simulink model "Acceleration_R2016a"  (Simulink 8.7)
settings: Solver=VariableStepAuto  SolverMode=SingleTasking  StartTime=0.0  StopTime=30  FixedStep=0.1  RelTol=1e-3
values from neighbouring files (symbols this model uses):
  a = 31.111    [variabeln.m]
  b = -12.44444    [variabeln.m]
  Fz0 = 400*g    (= 3924)    [variabeln.m]
  g = 9.81    [variabeln.m]
  gear_ratio = 7.13    [variabeln.m]
  h_CoM = 0.5    [variabeln.m]
  J = 1    [variabeln.m]
  K_lqr = lqr(A,B,Q,R)    [variabeln.m]
  l = l_f+l_r    (= 3)    [variabeln.m]
  l_f = 1.5    [variabeln.m]
  lambda_target = 0.1    [variabeln.m]
  m = 700    [variabeln.m]
  Q = 100    [variabeln.m]
  R = 0.01    [variabeln.m]
  r = 0.25    [variabeln.m]
  saturation_voltage_high = 4.9    [variabeln.m]
  saturation_voltage_low = 0.4    [variabeln.m]
  Ta0 = 800    [variabeln.m]
  theta1 = 0.86    [variabeln.m]
  theta2 = 33.82    [variabeln.m]
  theta3 = 0.35    [variabeln.m]
  W_luft = 0.5*cw*A*rho    (= 0.45)    [variabeln.m]
libraries: simulink x1
settings Model: Creator=frede  LastModifiedBy=Dominic
settings DataIOCC: ExternalInput=[t, u,m,g,r,J,theta1,theta2,theta3,v0,gear_ratio,v_max]  LimitDataPoints=off  SaveFormat=Dataset
settings DebuggingCC: UnderspecifiedInitializationDetection=Simplified  MergeDetectMultiDrivingBlocksExec=error  MaxConsecutiveZCsMsg=none  SFUnexpectedBacktrackingDiag=error  SFNoUnconditionalDefaultTransitionDiag=error
settings HardwareCC: ProdBitPerPointer=64  ProdLargestAtomicFloat=Float  ProdIntDivRoundTo=Zero  ProdEndianess=LittleEndian  ProdWordSize=64  ProdHWDeviceType=Intel->x86-64 (Windows64)
settings ModelReferenceCC: PropagateSignalLabelsOutOfModel=on
settings GRTTargetCC: TargetLangStandard=C99 (ISO)  GeneratePreprocessorConditionals=Use local settings
settings ConfigComp: CovMetricSettings=dwe  CovHtmlReporting=off  CovSaveCumulativeToWorkspaceVar=off  CovSaveSingleToWorkspaceVar=off  CovModelRefEnable=off  CovExternalEMLEnable=on

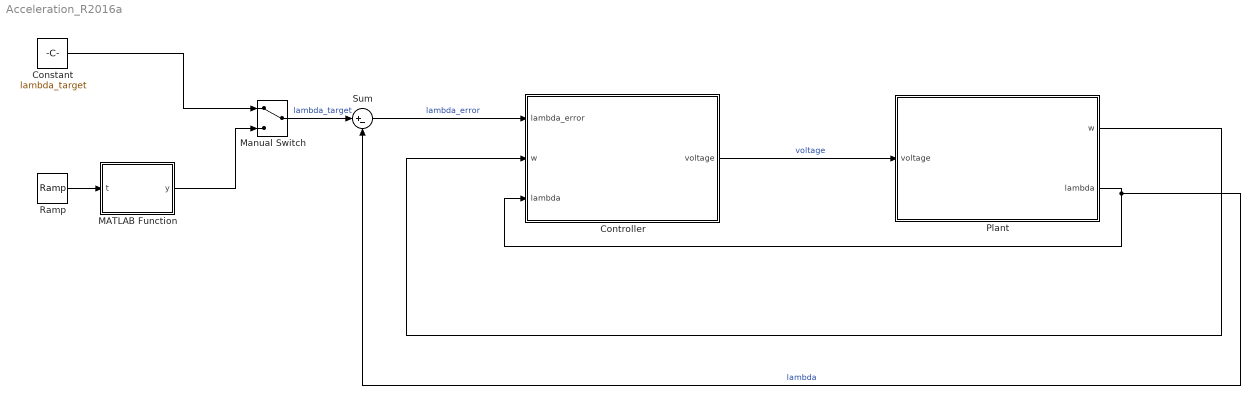
== system Acceleration_R2016a ==
  Constant : Constant  Value=lambda_target
  Controller : Subsystem
  MATLAB Function : MATLAB Function  TreatAsAtomicUnit=on
  Manual Switch : ManualSwitch
  Plant : Subsystem
  Ramp : simulink/Sources/Ramp  slope=1  start=0  X0=0
  Sum : Sum  Inputs=|+-
  wires:
  Sum/1 -> Controller/1(lambda_error)  "lambda_error"
  Ramp/1 -> MATLAB Function/1(t)
  MATLAB Function/1(y) -> Manual Switch/2
  Manual Switch/1 -> Sum/1  "lambda_target"
  Constant/1 -> Manual Switch/1
  Plant/2(lambda) -> Controller/3(lambda), Sum/2  "lambda"
  Controller/1(voltage) -> Plant/1(voltage)  "voltage"
  Plant/1(w) -> Controller/2(w)

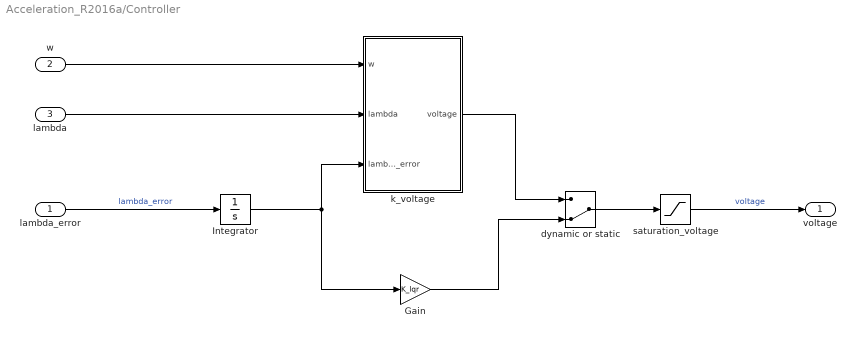
== system Acceleration_R2016a/Controller ==
  lambda_error : Inport
  w : Inport  Port=2
  lambda : Inport  Port=3
  Gain : Gain  Gain=K_lqr
  Integrator : Integrator
  dynamic or static : ManualSwitch  CurrentSetting=0
  k_voltage : MATLAB Function  TreatAsAtomicUnit=on
  saturation_voltage : Saturate  UpperLimit=saturation_voltage_high  LowerLimit=saturation_voltage_low
  voltage : Outport
  wires:
  saturation_voltage/1 -> voltage/1  "voltage"
  lambda_error/1 -> Integrator/1  "lambda_error"
  dynamic or static/1 -> saturation_voltage/1
  Gain/1 -> dynamic or static/2
  Integrator/1 -> k_voltage/3(lambda_error), Gain/1
  k_voltage/1(voltage) -> dynamic or static/1
  w/1 -> k_voltage/1(w)
  lambda/1 -> k_voltage/2(lambda)

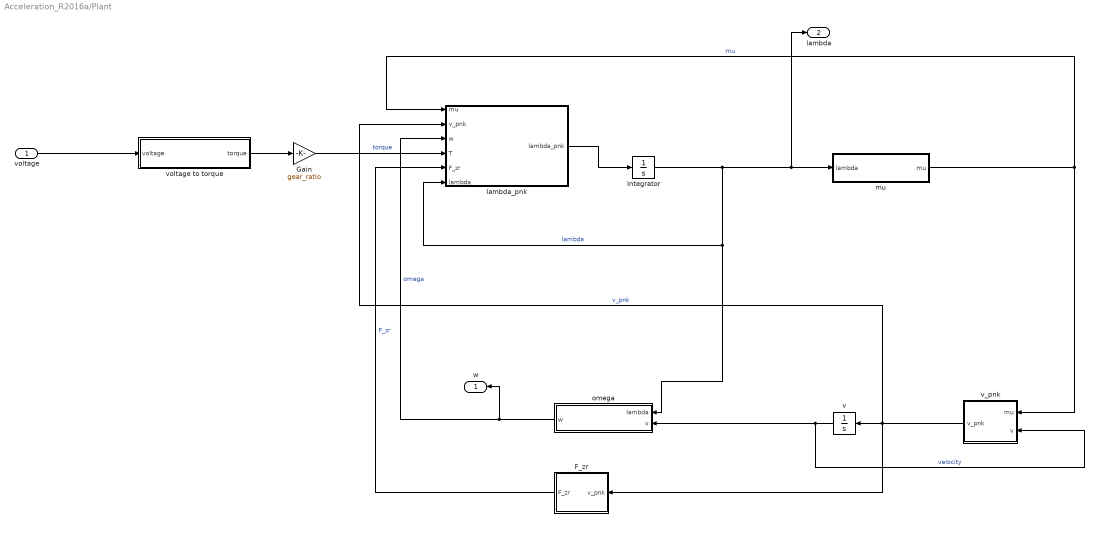
== system Acceleration_R2016a/Plant ==
  voltage : Inport
  F_zr : MATLAB Function  TreatAsAtomicUnit=on
  Gain : Gain  Gain=gear_ratio
  Integrator : Integrator
  lambda_pnk : MATLAB Function  TreatAsAtomicUnit=on
  mu : MATLAB Function  TreatAsAtomicUnit=on
  omega : MATLAB Function  TreatAsAtomicUnit=on
  v : Integrator  InitialCondition=0.1
  v_pnk : MATLAB Function  TreatAsAtomicUnit=on
  voltage to torque : MATLAB Function  TreatAsAtomicUnit=on
  w : Outport
  lambda : Outport  Port=2
  wires:
  Integrator/1 -> omega/1(lambda), lambda_pnk/6(lambda), lambda/1, mu/1(lambda)  "lambda"
  mu/1(mu) -> lambda_pnk/1(mu), v_pnk/1(mu)  "mu"
  v_pnk/1(v_pnk) -> lambda_pnk/2(v_pnk), v/1, F_zr/1(v_pnk)  "v_pnk"
  F_zr/1(F_zr) -> lambda_pnk/5(F_zr)  "F_zr"
  lambda_pnk/1(lambda_pnk) -> Integrator/1
  omega/1(w) -> w/1, lambda_pnk/3(w)  "omega"
  v/1 -> omega/2(v), v_pnk/2(v)  "velocity"
  voltage/1 -> voltage to torque/1(voltage)
  voltage to torque/1(torque) -> Gain/1
  Gain/1 -> lambda_pnk/4(T)  "torque"

== matlab function Plant/mu ==
  data: lambda input double; mu output double; theta1 parameter double; theta2 parameter double; theta3 parameter double
function mu = mu(lambda, theta1, theta2, theta3)

if lambda>=0
    mu = theta1*(1-exp(-theta2*lambda))-lambda*theta3;
    
else
         mu = -(theta1*(1-exp(-theta2*abs(lambda)))-abs(lambda)*theta3);


end

== matlab function MATLAB Function ==
  data: y output double; t input double; lambda_target parameter double
function y = lambda_target(t, lambda_target)

y = lambda_target*exp(-0.1*t);
end

== matlab function Plant/F_zr ==
  data: F_zr output double; v_pnk input double; m parameter double; h_CoM parameter double; l parameter double; g parameter double; l_f parameter double
function F_zr = fcn(v_pnk,m, h_CoM, l, g, l_f)

F_zr=m*h_CoM/l*v_pnk+m*g*l_f/l;

end

== matlab function Plant/lambda_pnk ==
  data: mu input double; v_pnk input double; lambda_pnk output double; w input double; T input double; F_zr input double; r parameter double; J parameter double; lambda input double
function lambda_pnk = fcn(mu,v_pnk,w,T,F_zr, r, J,lambda)

lambda_pnk=-v_pnk/(w*r)+(1-lambda)/w*T/J-(1-lambda)/w*r*F_zr*mu/J;

end

== matlab function Plant/omega ==
  data: lambda input double; v input double; w output double; r parameter double
function w = fcn(lambda, v,r)

w=v/(1-lambda)/r;

end

== matlab function Plant/v_pnk ==
  data: mu input double; v_pnk output double; g parameter double; l_f parameter double; l parameter double; h_CoM parameter double; v input double; W_luft parameter double; m parameter double
function v_pnk = fcn(mu,g, l_f, l, h_CoM,v,W_luft, m)

v_pnk=mu*g*l_f/(l-mu*h_CoM)-W_luft/((1-h_CoM/l*mu)*m)*v^2;

end

== matlab function Plant/voltage to torque ==
  data: voltage input double; torque output double; a parameter double; b parameter double
function torque = fcn(voltage,a, b)

torque = a*voltage+b;

== matlab function Controller/k_voltage ==
  data: voltage output double; w input double; lambda input double; m parameter double; r parameter double; J parameter double; theta1 parameter double; theta2 parameter double; theta3 parameter double; R parameter double; Q parameter double; lambda_error input double; Ta0 parameter double; Fz0 parameter double; a parameter double; b parameter double
function voltage = fcn(w,lambda,m, r, J, theta1, theta2, theta3, R, Q,lambda_error, Ta0, Fz0, a, b)



A1=Ta0/(J*w)-Fz0*r/(J*w)*(theta1*theta2*exp(-lambda*theta2)-theta3)+Fz0*r/(J*w)*(theta1*(1-exp(-lambda*theta2)-lambda*theta2*exp(-lambda*theta2))-2*lambda*theta3)-Fz0/(m*r*w)*(theta1*theta2*exp(-lambda*theta2)-theta3);

B1=1/(J*w)-lambda/(J*w);


    voltage_before = lambda_error*(A1+B1*sqrt(A1^2+B1^2*Q/R))/B1;


    voltage = voltage_before+(Ta0-b)/a; % dvoltage+voltage
 

end
